simulink model "exp_6"  (R2013b)
settings: Solver=ode3  StartTime=0.0  StopTime=10.0  FixedStep=0.02  RelTol=1e-3
libraries: simulink x1
settings Model: Creator=lenovo  LastModifiedBy=lenovo

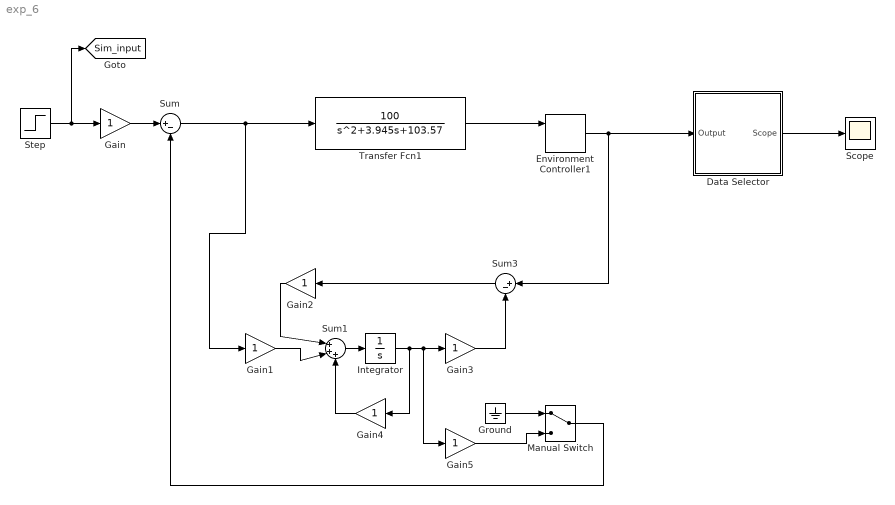
== system exp_6 ==
  "Data Selector " : Subsystem
  Environment Controller1 : simulink/Signal Routing/Environment Controller
  Gain{,1..5} (6 alike) : Gain
  Ground : Ground
  Integrator : Integrator
  Manual Switch : ManualSwitch
  Scope : Scope
  Step : Step  SampleTime=0
  Sum : Sum  Inputs=|+-
  Sum1 : Sum  Inputs=|+++
  Sum3 : Sum  Inputs=|+-
  Transfer Fcn1 : TransferFcn  Numerator=[100]  Denominator=[1 3.945 103.57]
  tag scope: Sim_input=global
  wires:
  Step/1 -> [Sim_input], Gain/1
  Gain/1 -> Sum/1
  Sum/1 -> Gain1/1, Transfer Fcn1/1
  Transfer Fcn1/1 -> Environment Controller1/1
  Sum3/1 -> Gain2/1
  Gain2/1 -> Sum1/1
  Gain1/1 -> Sum1/2
  Sum1/1 -> Integrator/1
  Integrator/1 -> Gain4/1, Gain5/1, Gain3/1
  Gain3/1 -> Sum3/2
  Gain4/1 -> Sum1/3
  Ground/1 -> Manual Switch/1
  Gain5/1 -> Manual Switch/2
  Manual Switch/1 -> Sum/2
  Environment Controller1/1 -> Sum3/1, "Data Selector "/1(Output)
  "Data Selector "/1(Scope) -> Scope/1

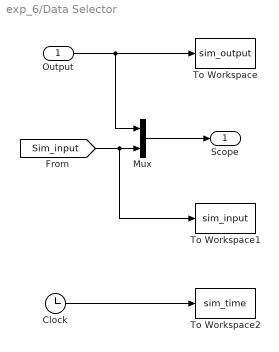
== system exp_6/Data Selector  ==
  Output : Inport
  Clock : Clock
  Mux : Mux  Inputs=2
  To Workspace : ToWorkspace  VariableName=sim_output  SampleTime=-1  SaveFormat=Timeseries
  To Workspace1 : ToWorkspace  VariableName=sim_input  SampleTime=-1  SaveFormat=Timeseries
  To Workspace2 : ToWorkspace  VariableName=sim_time  SampleTime=-1  SaveFormat=Timeseries
  Scope : Outport
  wires:
  Output/1 -> Mux/1, To Workspace/1
  [Sim_input] -> To Workspace1/1, Mux/2
  Mux/1 -> Scope/1
  Clock/1 -> To Workspace2/1
